simulink model "FourWheelSim_base"  (R2021b)
settings: Solver=ode4  StartTime=0.0  StopTime=100  FixedStep=0.001  EnableMultiTasking=on
values from neighbouring files (symbols this model uses):
  a_f = [1.434106444513048,-3.490394354141787e-04,2.761516722659314,6.000050177239062e+04,2.990012596710455e+03,-1.736376596503330e-04,0.526021936511837]    [VehicleParams20_ver230707.m]
  a_r = a_f    [VehicleParams20_ver230707.m]
  afx_f = [1.736519934348130,-2.903281841026900e-04,2.651682004580759,7.000047010028531e+04,3.270011055825476e+03,-0.001252141095807,1.596836353939939]    [VehicleParams20_ver230707.m]
  afx_r = afx_f    [VehicleParams20_ver230707.m]
  agx_f = [0.230000000000000,2.936116597489246e+04,7.137436879966481e+03,0,0]    [VehicleParams20_ver230707.m]
  agx_r = agx_f    [VehicleParams20_ver230707.m]
  agy_f = [0.852564208514954,3.000069064154418e+04,2.070023877794581e+03,-5.089267464508360e-04,0.519364283925805]    [VehicleParams20_ver230707.m]
  agy_r = agy_f    [VehicleParams20_ver230707.m]
  b_f = [3.436650779629654,1.566044221042620e-05,0.028598122547093,3.408741969645286e+03,5.995144285148312e+03,-1.736376595720277e-04,0.526021936449385]    [VehicleParams20_ver230707.m]
  Brake_Factor = 0.66    [VehicleParams20_ver230707.m]
  Cd = Cd/(40/3.6)^2    (= 0.6885)    [VehicleParams20_ver230707.m]
  CLF = DFf/40/40    (= 0.06)    [VehicleParams20_ver230707.m]
  CLR = DFr/40/40    (= 0.065)    [VehicleParams20_ver230707.m]
  cPiston_Area_F = 2*pi*(0.0254/2)^2    (= 0.00101341495819)    [VehicleParams20_ver230707.m]
  cPiston_Area_R = 2*pi*(0.0254/2)^2    (= 0.00101341495819)    [VehicleParams20_ver230707.m]
  delta = 15.5    [VehicleParams20_ver230707.m]
  df = 1.225    [VehicleParams20_ver230707.m]
  dr = 1.225    [VehicleParams20_ver230707.m]
  eff_Radius_F = (180/2-13.5)/1000    (= 0.0765)    [VehicleParams20_ver230707.m]
  eff_Radius_R = (180/2-13.5)/1000    (= 0.0765)    [VehicleParams20_ver230707.m]
  Fd = 60*2    (= 120)    [VehicleParams20_ver230707.m]
  Frtoe = 0    [VehicleParams20_ver230707.m]
  gear_f = 13.75    [VehicleParams20_ver230707.m]
  gear_r = 13.75    [VehicleParams20_ver230707.m]
  hg = 0.28    [VehicleParams20_ver230707.m]
  HV_voltage = 600    [VehicleParams20_ver230707.m]
  I = 112    [VehicleParams20_ver230707.m]
  ini_v = ini_speed/3.6    (= 10.4166666667)    [VehicleParams20_ver230707.m]
  Kframe = 5.94*10^6    (= 5940000)    [VehicleParams20_ver230707.m]
  kk_f = 2800*180/pi    (= 160428.182637)    [VehicleParams20_ver230707.m]
  kk_r = 4200*180/pi    (= 240642.273955)    [VehicleParams20_ver230707.m]
  krfr = 0.5    [VehicleParams20_ver230707.m]
  l = 1.530    (= 1.53)    [VehicleParams20_ver230707.m]
  lf = l*(1-WBf)    (= 0.7956)    [VehicleParams20_ver230707.m]
  lr = l*WBf    (= 0.7344)    [VehicleParams20_ver230707.m]
  M = 200+60    (= 260)    [VehicleParams20_ver230707.m]
  mu_tire_F = 0.587-0.587+0.55    (= 0.55)    [VehicleParams20_ver230707.m]
  mu_tire_R = 0.587-0.587+0.55    (= 0.55)    [VehicleParams20_ver230707.m]
  Mwf = Iwf/Rwf/Rwf    (= 3.82716814816)    [VehicleParams20_ver230707.m]
  Mwr = Iwr/Rwr/Rwr    (= 3.82716814816)    [VehicleParams20_ver230707.m]
  rcf = 0.000    (= 0)    [VehicleParams20_ver230707.m]
  rch = rcf*WBf+rcr*(1-WBf)    (= 0)    [VehicleParams20_ver230707.m]
  rcr = 0.000    (= 0)    [VehicleParams20_ver230707.m]
  Reartoe = -2    [VehicleParams20_ver230707.m]
  Rr_toe = Reartoe*pi/180    (= -0.0349065850399)    [VehicleParams20_ver230707.m]
  Rwf = 18*(25.4/1000)/2    (= 0.2286)    [VehicleParams20_ver230707.m]
  Rwr = 18*(25.4/1000)/2    (= 0.2286)    [VehicleParams20_ver230707.m]
  T_TireF = TireL_f/V    (= 0.036760000032)    [VehicleParams20_ver230707.m]
  T_TireR = TireL_r/V    (= 0.036760000032)    [VehicleParams20_ver230707.m]
  tspeed = 37.5    [VehicleParams20_ver230707.m]
  WBf = 0.48    [VehicleParams20_ver230707.m]
  zc_f = castrail_Fr/1000    (= 0)    [VehicleParams20_ver230707.m]
  zc_r = castrail_Rr/1000    (= 0)    [VehicleParams20_ver230707.m]
libraries: simulink x25, dspstat3 x1
(part 3 of 4)

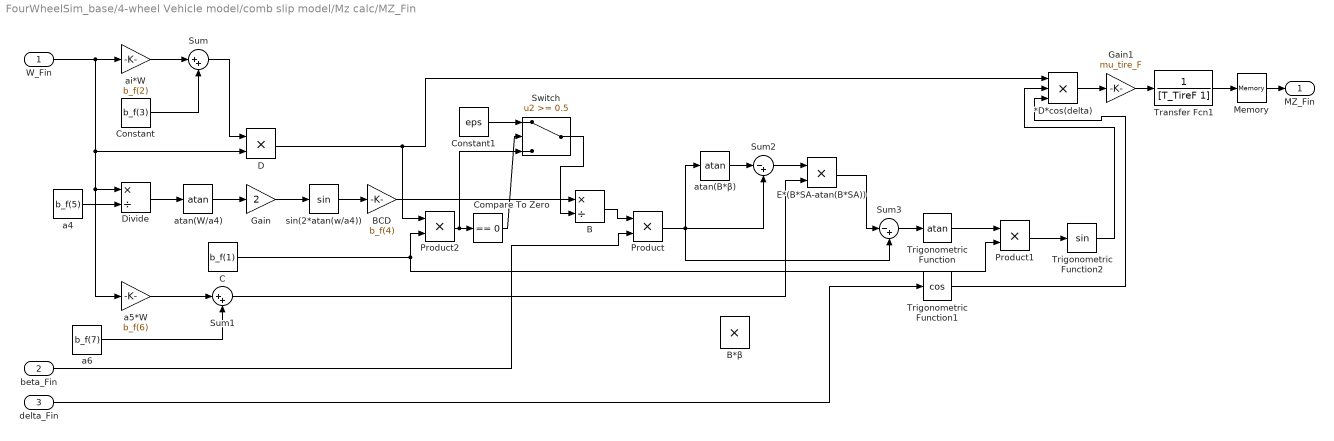
== system FourWheelSim_base/4-wheel Vehicle model/comb slip model/Mz calc/MZ_Fin ==
  W_Fin : Inport
  beta_Fin : Inport  Port=2
  delta_Fin : Inport  Port=3
  *D*cos(delta) : Product  Inputs=3  RndMeth=Zero
  B : Product  Inputs=*/
  B*β : Product  Inputs=**
  BCD : Gain  Gain=b_f(4)
  C : Constant  Value=b_f(1)
  Compare To Zero : simulink/Logic and Bit Operations/Compare To Zero  relop===  OutDataTypeStr=boolean
  Constant : Constant  Value=b_f(3)
  Constant1 : Constant  Value=eps
  D : Product  RndMeth=Zero
  Divide : Product  Inputs=*/
  E*(B*SA-atan(B*SA)) : Product  RndMeth=Zero
  Gain : Gain  Gain=2
  Gain1 : Gain  Gain=mu_tire_F
  Memory : Memory
  Product : Product  RndMeth=Zero
  Product1 : Product  RndMeth=Zero
  Product2 : Product
  Sum : Sum  Inputs=|++
  Sum1 : Sum  Inputs=|++
  Sum2 : Sum  Inputs=|-+
  Sum3 : Sum  Inputs=|-+
  Switch : Switch  Threshold=0.5
  Transfer Fcn1 : TransferFcn  Denominator=[T_TireF 1]
  Trigonometric Function : Trigonometry  Operator=atan
  Trigonometric Function1 : Trigonometry  Operator=cos
  Trigonometric Function2 : Trigonometry
  a4 : Constant  Value=b_f(5)
  a5*W : Gain  Gain=b_f(6)
  a6 : Constant  Value=b_f(7)
  ai*W : Gain  Gain=b_f(2)
  atan(B*β) : Trigonometry  Operator=atan
  atan(W/a4) : Trigonometry  Operator=atan
  sin(2*atan(w/a4)) : Trigonometry
  MZ_Fin : Outport  VectorParamsAs1DForOutWhenUnconnected=off
  wires:
  Constant/1 -> Sum/2
  ai*W/1 -> Sum/1
  Sum/1 -> D/1
  a4/1 -> Divide/2
  Divide/1 -> atan(W/a4)/1
  atan(W/a4)/1 -> Gain/1
  Gain/1 -> sin(2*atan(w/a4))/1
  sin(2*atan(w/a4))/1 -> BCD/1
  BCD/1 -> B/1
  C/1 -> Product1/2, Product2/2
  a5*W/1 -> Sum1/1
  a6/1 -> Sum1/2
  B/1 -> Product/1
  beta_Fin/1 -> Product/2
  Sum1/1 -> E*(B*SA-atan(B*SA))/2
  Sum3/1 -> Trigonometric Function/1
  D/1 -> Product2/1, *D*cos(delta)/1
  Gain1/1 -> Transfer Fcn1/1
  delta_Fin/1 -> Trigonometric Function1/1
  Trigonometric Function1/1 -> *D*cos(delta)/3
  Trigonometric Function/1 -> Product1/1
  Trigonometric Function2/1 -> *D*cos(delta)/2
  Product1/1 -> Trigonometric Function2/1
  W_Fin/1 -> a5*W/1, Divide/1, D/2, ai*W/1
  Product2/1 -> Switch/3, Compare To Zero/1
  Compare To Zero/1 -> Switch/2
  Constant1/1 -> Switch/1
  Switch/1 -> B/2
  *D*cos(delta)/1 -> Gain1/1
  Transfer Fcn1/1 -> Memory/1
  Memory/1 -> MZ_Fin/1
  Product/1 -> Sum2/2, Sum3/2, atan(B*β)/1
  atan(B*β)/1 -> Sum2/1
  Sum2/1 -> E*(B*SA-atan(B*SA))/1
  E*(B*SA-atan(B*SA))/1 -> Sum3/1

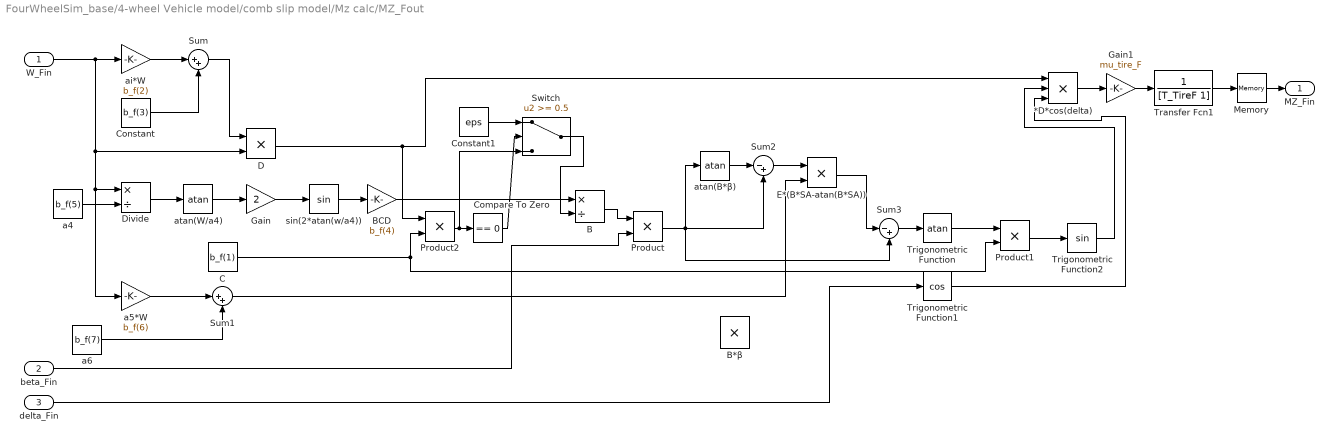
== system FourWheelSim_base/4-wheel Vehicle model/comb slip model/Mz calc/MZ_Fout ==
  W_Fin : Inport
  beta_Fin : Inport  Port=2
  delta_Fin : Inport  Port=3
  *D*cos(delta) : Product  Inputs=3  RndMeth=Zero
  B : Product  Inputs=*/
  B*β : Product  Inputs=**
  BCD : Gain  Gain=b_f(4)
  C : Constant  Value=b_f(1)
  Compare To Zero : simulink/Logic and Bit Operations/Compare To Zero  relop===  OutDataTypeStr=boolean
  Constant : Constant  Value=b_f(3)
  Constant1 : Constant  Value=eps
  D : Product  RndMeth=Zero
  Divide : Product  Inputs=*/
  E*(B*SA-atan(B*SA)) : Product  RndMeth=Zero
  Gain : Gain  Gain=2
  Gain1 : Gain  Gain=mu_tire_F
  Memory : Memory
  Product : Product  RndMeth=Zero
  Product1 : Product  RndMeth=Zero
  Product2 : Product
  Sum : Sum  Inputs=|++
  Sum1 : Sum  Inputs=|++
  Sum2 : Sum  Inputs=|-+
  Sum3 : Sum  Inputs=|-+
  Switch : Switch  Threshold=0.5
  Transfer Fcn1 : TransferFcn  Denominator=[T_TireF 1]
  Trigonometric Function : Trigonometry  Operator=atan
  Trigonometric Function1 : Trigonometry  Operator=cos
  Trigonometric Function2 : Trigonometry
  a4 : Constant  Value=b_f(5)
  a5*W : Gain  Gain=b_f(6)
  a6 : Constant  Value=b_f(7)
  ai*W : Gain  Gain=b_f(2)
  atan(B*β) : Trigonometry  Operator=atan
  atan(W/a4) : Trigonometry  Operator=atan
  sin(2*atan(w/a4)) : Trigonometry
  MZ_Fin : Outport  VectorParamsAs1DForOutWhenUnconnected=off
  wires:
  Constant/1 -> Sum/2
  ai*W/1 -> Sum/1
  Sum/1 -> D/1
  a4/1 -> Divide/2
  Divide/1 -> atan(W/a4)/1
  atan(W/a4)/1 -> Gain/1
  Gain/1 -> sin(2*atan(w/a4))/1
  sin(2*atan(w/a4))/1 -> BCD/1
  BCD/1 -> B/1
  C/1 -> Product1/2, Product2/2
  a5*W/1 -> Sum1/1
  a6/1 -> Sum1/2
  B/1 -> Product/1
  beta_Fin/1 -> Product/2
  Sum1/1 -> E*(B*SA-atan(B*SA))/2
  Sum3/1 -> Trigonometric Function/1
  D/1 -> Product2/1, *D*cos(delta)/1
  Gain1/1 -> Transfer Fcn1/1
  delta_Fin/1 -> Trigonometric Function1/1
  Trigonometric Function1/1 -> *D*cos(delta)/3
  Trigonometric Function/1 -> Product1/1
  Trigonometric Function2/1 -> *D*cos(delta)/2
  Product1/1 -> Trigonometric Function2/1
  W_Fin/1 -> a5*W/1, Divide/1, D/2, ai*W/1
  Product2/1 -> Switch/3, Compare To Zero/1
  Compare To Zero/1 -> Switch/2
  Constant1/1 -> Switch/1
  Switch/1 -> B/2
  *D*cos(delta)/1 -> Gain1/1
  Transfer Fcn1/1 -> Memory/1
  Memory/1 -> MZ_Fin/1
  Product/1 -> Sum2/2, Sum3/2, atan(B*β)/1
  atan(B*β)/1 -> Sum2/1
  Sum2/1 -> E*(B*SA-atan(B*SA))/1
  E*(B*SA-atan(B*SA))/1 -> Sum3/1

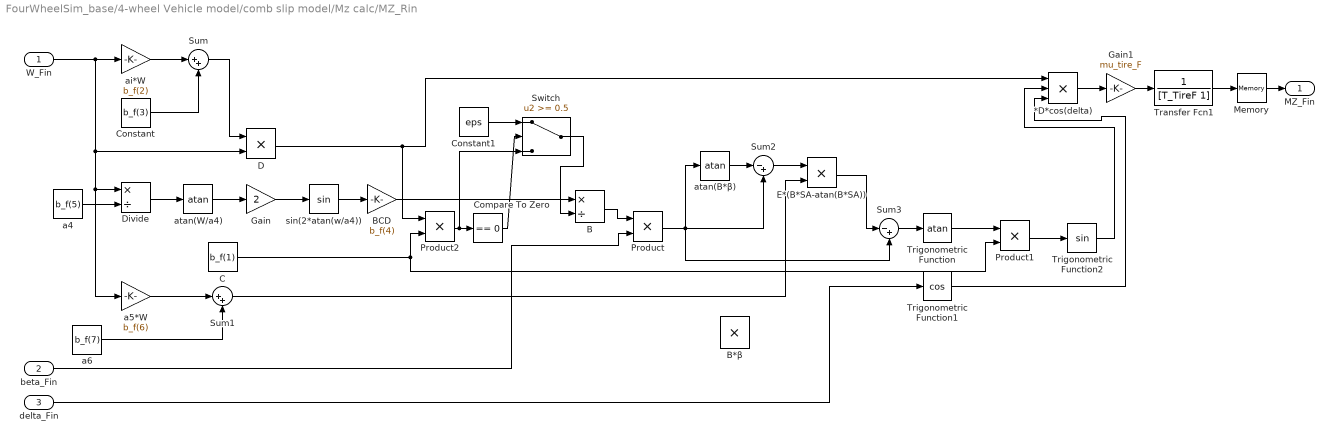
== system FourWheelSim_base/4-wheel Vehicle model/comb slip model/Mz calc/MZ_Rin ==
  W_Fin : Inport
  beta_Fin : Inport  Port=2
  delta_Fin : Inport  Port=3
  *D*cos(delta) : Product  Inputs=3  RndMeth=Zero
  B : Product  Inputs=*/
  B*β : Product  Inputs=**
  BCD : Gain  Gain=b_f(4)
  C : Constant  Value=b_f(1)
  Compare To Zero : simulink/Logic and Bit Operations/Compare To Zero  relop===  OutDataTypeStr=boolean
  Constant : Constant  Value=b_f(3)
  Constant1 : Constant  Value=eps
  D : Product  RndMeth=Zero
  Divide : Product  Inputs=*/
  E*(B*SA-atan(B*SA)) : Product  RndMeth=Zero
  Gain : Gain  Gain=2
  Gain1 : Gain  Gain=mu_tire_F
  Memory : Memory
  Product : Product  RndMeth=Zero
  Product1 : Product  RndMeth=Zero
  Product2 : Product
  Sum : Sum  Inputs=|++
  Sum1 : Sum  Inputs=|++
  Sum2 : Sum  Inputs=|-+
  Sum3 : Sum  Inputs=|-+
  Switch : Switch  Threshold=0.5
  Transfer Fcn1 : TransferFcn  Denominator=[T_TireF 1]
  Trigonometric Function : Trigonometry  Operator=atan
  Trigonometric Function1 : Trigonometry  Operator=cos
  Trigonometric Function2 : Trigonometry
  a4 : Constant  Value=b_f(5)
  a5*W : Gain  Gain=b_f(6)
  a6 : Constant  Value=b_f(7)
  ai*W : Gain  Gain=b_f(2)
  atan(B*β) : Trigonometry  Operator=atan
  atan(W/a4) : Trigonometry  Operator=atan
  sin(2*atan(w/a4)) : Trigonometry
  MZ_Fin : Outport  VectorParamsAs1DForOutWhenUnconnected=off
  wires:
  Constant/1 -> Sum/2
  ai*W/1 -> Sum/1
  Sum/1 -> D/1
  a4/1 -> Divide/2
  Divide/1 -> atan(W/a4)/1
  atan(W/a4)/1 -> Gain/1
  Gain/1 -> sin(2*atan(w/a4))/1
  sin(2*atan(w/a4))/1 -> BCD/1
  BCD/1 -> B/1
  C/1 -> Product1/2, Product2/2
  a5*W/1 -> Sum1/1
  a6/1 -> Sum1/2
  B/1 -> Product/1
  beta_Fin/1 -> Product/2
  Sum1/1 -> E*(B*SA-atan(B*SA))/2
  Sum3/1 -> Trigonometric Function/1
  D/1 -> Product2/1, *D*cos(delta)/1
  Gain1/1 -> Transfer Fcn1/1
  delta_Fin/1 -> Trigonometric Function1/1
  Trigonometric Function1/1 -> *D*cos(delta)/3
  Trigonometric Function/1 -> Product1/1
  Trigonometric Function2/1 -> *D*cos(delta)/2
  Product1/1 -> Trigonometric Function2/1
  W_Fin/1 -> a5*W/1, Divide/1, D/2, ai*W/1
  Product2/1 -> Switch/3, Compare To Zero/1
  Compare To Zero/1 -> Switch/2
  Constant1/1 -> Switch/1
  Switch/1 -> B/2
  *D*cos(delta)/1 -> Gain1/1
  Transfer Fcn1/1 -> Memory/1
  Memory/1 -> MZ_Fin/1
  Product/1 -> Sum2/2, Sum3/2, atan(B*β)/1
  atan(B*β)/1 -> Sum2/1
  Sum2/1 -> E*(B*SA-atan(B*SA))/1
  E*(B*SA-atan(B*SA))/1 -> Sum3/1

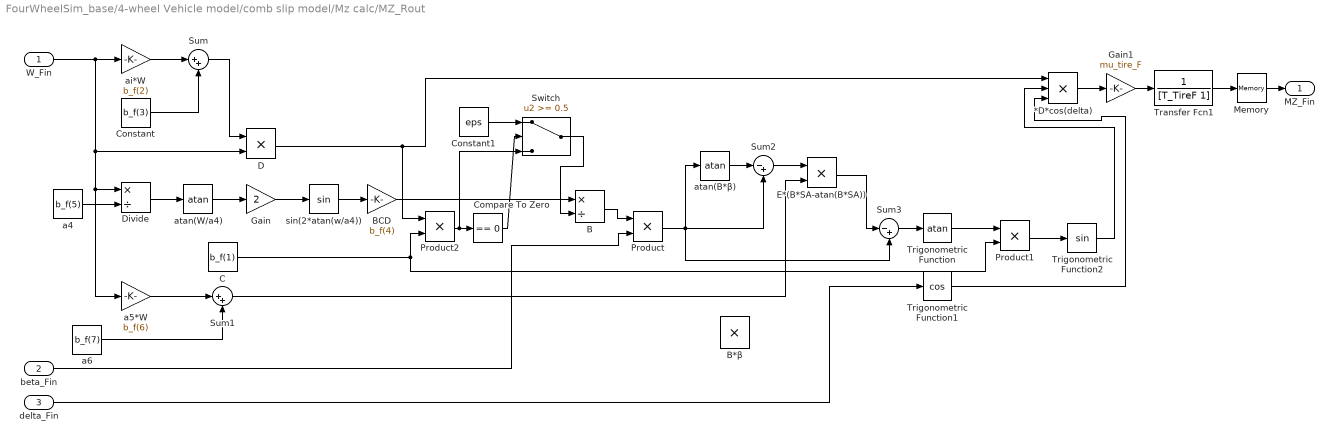
== system FourWheelSim_base/4-wheel Vehicle model/comb slip model/Mz calc/MZ_Rout ==
  W_Fin : Inport
  beta_Fin : Inport  Port=2
  delta_Fin : Inport  Port=3
  *D*cos(delta) : Product  Inputs=3  RndMeth=Zero
  B : Product  Inputs=*/
  B*β : Product  Inputs=**
  BCD : Gain  Gain=b_f(4)
  C : Constant  Value=b_f(1)
  Compare To Zero : simulink/Logic and Bit Operations/Compare To Zero  relop===  OutDataTypeStr=boolean
  Constant : Constant  Value=b_f(3)
  Constant1 : Constant  Value=eps
  D : Product  RndMeth=Zero
  Divide : Product  Inputs=*/
  E*(B*SA-atan(B*SA)) : Product  RndMeth=Zero
  Gain : Gain  Gain=2
  Gain1 : Gain  Gain=mu_tire_F
  Memory : Memory
  Product : Product  RndMeth=Zero
  Product1 : Product  RndMeth=Zero
  Product2 : Product
  Sum : Sum  Inputs=|++
  Sum1 : Sum  Inputs=|++
  Sum2 : Sum  Inputs=|-+
  Sum3 : Sum  Inputs=|-+
  Switch : Switch  Threshold=0.5
  Transfer Fcn1 : TransferFcn  Denominator=[T_TireF 1]
  Trigonometric Function : Trigonometry  Operator=atan
  Trigonometric Function1 : Trigonometry  Operator=cos
  Trigonometric Function2 : Trigonometry
  a4 : Constant  Value=b_f(5)
  a5*W : Gain  Gain=b_f(6)
  a6 : Constant  Value=b_f(7)
  ai*W : Gain  Gain=b_f(2)
  atan(B*β) : Trigonometry  Operator=atan
  atan(W/a4) : Trigonometry  Operator=atan
  sin(2*atan(w/a4)) : Trigonometry
  MZ_Fin : Outport  VectorParamsAs1DForOutWhenUnconnected=off
  wires:
  Constant/1 -> Sum/2
  ai*W/1 -> Sum/1
  Sum/1 -> D/1
  a4/1 -> Divide/2
  Divide/1 -> atan(W/a4)/1
  atan(W/a4)/1 -> Gain/1
  Gain/1 -> sin(2*atan(w/a4))/1
  sin(2*atan(w/a4))/1 -> BCD/1
  BCD/1 -> B/1
  C/1 -> Product1/2, Product2/2
  a5*W/1 -> Sum1/1
  a6/1 -> Sum1/2
  B/1 -> Product/1
  beta_Fin/1 -> Product/2
  Sum1/1 -> E*(B*SA-atan(B*SA))/2
  Sum3/1 -> Trigonometric Function/1
  D/1 -> Product2/1, *D*cos(delta)/1
  Gain1/1 -> Transfer Fcn1/1
  delta_Fin/1 -> Trigonometric Function1/1
  Trigonometric Function1/1 -> *D*cos(delta)/3
  Trigonometric Function/1 -> Product1/1
  Trigonometric Function2/1 -> *D*cos(delta)/2
  Product1/1 -> Trigonometric Function2/1
  W_Fin/1 -> a5*W/1, Divide/1, D/2, ai*W/1
  Product2/1 -> Switch/3, Compare To Zero/1
  Compare To Zero/1 -> Switch/2
  Constant1/1 -> Switch/1
  Switch/1 -> B/2
  *D*cos(delta)/1 -> Gain1/1
  Transfer Fcn1/1 -> Memory/1
  Memory/1 -> MZ_Fin/1
  Product/1 -> Sum2/2, Sum3/2, atan(B*β)/1
  atan(B*β)/1 -> Sum2/1
  Sum2/1 -> E*(B*SA-atan(B*SA))/1
  E*(B*SA-atan(B*SA))/1 -> Sum3/1

== system FourWheelSim_base/4-wheel Vehicle model/comb slip model/comb Fx calc/Force_Fin_comb_FX ==
  W_Fin : Inport
  beta_Fin : Inport  Port=2
  slip rate : Inport  Port=3
  *D : Product  RndMeth=Zero
  B : Product  Inputs=*/
  BCD : Gain  Gain=agx_f(2)
  C : Constant  Value=agx_f(1)
  Compare To Zero : simulink/Logic and Bit Operations/Compare To Zero  relop===  OutDataTypeStr=boolean
  Constant1 : Constant  Value=eps
  Divide : Product  Inputs=*/
  E*(B*SA-atan(B*SA)) : Product  RndMeth=Zero
  Gain : Gain  Gain=2
  Gain1 : Gain  Gain=mu_tire_F
  Product : Product  RndMeth=Zero
  Product1 : Product  RndMeth=Zero
  Product2 : Product
  Scope : Scope
  Sum1 : Sum  Inputs=|++
  Sum2 : Sum  Inputs=|-+
  Sum3 : Sum  Inputs=|-+
  Switch : Switch  Threshold=0.5
  Tire Force : Subsystem
  Trigonometric Function : Trigonometry  Operator=atan
  Trigonometric Function2 : Trigonometry  Operator=cos
  a4 : Constant  Value=agx_f(3)
  a5*W : Gain  Gain=agy_f(4)
  a6 : Constant  Value=agx_f(5)
  atan(B*β) : Trigonometry  Operator=atan
  atan(W/a4) : Trigonometry  Operator=atan
  sin(2*atan(w/a4)) : Trigonometry
  Force_Fin : Outport  VectorParamsAs1DForOutWhenUnconnected=off
  wires:
  a4/1 -> Divide/2
  Divide/1 -> atan(W/a4)/1
  atan(W/a4)/1 -> Gain/1
  Gain/1 -> sin(2*atan(w/a4))/1
  sin(2*atan(w/a4))/1 -> BCD/1
  C/1 -> Product1/2, Product2/2
  a5*W/1 -> Sum1/1
  a6/1 -> Sum1/2
  B/1 -> Product/1
  Sum1/1 -> E*(B*SA-atan(B*SA))/2
  Sum3/1 -> Trigonometric Function/1
  Trigonometric Function/1 -> Product1/1
  Trigonometric Function2/1 -> *D/2
  Product1/1 -> Trigonometric Function2/1
  W_Fin/1 -> Tire Force/1(Load), Scope/1, a5*W/1, Divide/1
  *D/1 -> Gain1/1
  Gain1/1 -> Force_Fin/1
  Product/1 -> Sum2/2, Sum3/2, atan(B*β)/1
  atan(B*β)/1 -> Sum2/1
  Sum2/1 -> E*(B*SA-atan(B*SA))/1
  E*(B*SA-atan(B*SA))/1 -> Sum3/1
  Tire Force/1(Force_Rear) -> Product2/1, *D/1
  Product2/1 -> Switch/3, Compare To Zero/1
  Constant1/1 -> Switch/1
  Switch/1 -> B/2
  Compare To Zero/1 -> Switch/2
  BCD/1 -> B/1
  slip rate/1 -> Tire Force/2(Slip Rate)
  beta_Fin/1 -> Product/2

== system FourWheelSim_base/4-wheel Vehicle model/comb slip model/comb Fx calc/Force_Fout_comb_FX ==
  W_Fout : Inport
  beta_Fout : Inport  Port=2
  slip rate : Inport  Port=3
  *D : Product  RndMeth=Zero
  B : Product  Inputs=*/
  BCD : Gain  Gain=agx_f(2)
  C : Constant  Value=agx_f(1)
  Compare To Zero : simulink/Logic and Bit Operations/Compare To Zero  relop===  OutDataTypeStr=boolean
  Constant1 : Constant  Value=eps
  Divide : Product  Inputs=*/
  E*(B*SA-atan(B*SA)) : Product  RndMeth=Zero
  Gain : Gain  Gain=2
  Gain1 : Gain  Gain=mu_tire_F
  Product : Product  RndMeth=Zero
  Product1 : Product  RndMeth=Zero
  Product2 : Product
  Sum1 : Sum  Inputs=|++
  Sum2 : Sum  Inputs=|-+
  Sum3 : Sum  Inputs=|-+
  Switch : Switch  Threshold=0.5
  Tire Force : Subsystem
  Trigonometric Function : Trigonometry  Operator=atan
  Trigonometric Function2 : Trigonometry  Operator=cos
  a4 : Constant  Value=agx_f(3)
  a5*W : Gain  Gain=agy_f(4)
  a6 : Constant  Value=agx_f(5)
  atan(B*β) : Trigonometry  Operator=atan
  atan(W/a4) : Trigonometry  Operator=atan
  sin(2*atan(w/a4)) : Trigonometry
  Force_Fout : Outport  VectorParamsAs1DForOutWhenUnconnected=off
  wires:
  a4/1 -> Divide/2
  Divide/1 -> atan(W/a4)/1
  atan(W/a4)/1 -> Gain/1
  Gain/1 -> sin(2*atan(w/a4))/1
  sin(2*atan(w/a4))/1 -> BCD/1
  C/1 -> Product1/2, Product2/2
  a5*W/1 -> Sum1/1
  a6/1 -> Sum1/2
  B/1 -> Product/1
  Sum1/1 -> E*(B*SA-atan(B*SA))/2
  Sum3/1 -> Trigonometric Function/1
  Trigonometric Function/1 -> Product1/1
  Trigonometric Function2/1 -> *D/2
  Product1/1 -> Trigonometric Function2/1
  W_Fout/1 -> Tire Force/1(Load), a5*W/1, Divide/1
  *D/1 -> Gain1/1
  Product/1 -> Sum2/2, Sum3/2, atan(B*β)/1
  atan(B*β)/1 -> Sum2/1
  Sum2/1 -> E*(B*SA-atan(B*SA))/1
  E*(B*SA-atan(B*SA))/1 -> Sum3/1
  Tire Force/1(Force_Rear) -> Product2/1, *D/1
  Product2/1 -> Switch/3, Compare To Zero/1
  Constant1/1 -> Switch/1
  Switch/1 -> B/2
  Compare To Zero/1 -> Switch/2
  BCD/1 -> B/1
  slip rate/1 -> Tire Force/2(Slip Rate)
  beta_Fout/1 -> Product/2
  Gain1/1 -> Force_Fout/1

== system FourWheelSim_base/4-wheel Vehicle model/comb slip model/comb Fx calc/Force_Rin_comb_FX ==
  W_Rin : Inport
  beta_Rin : Inport  Port=2
  slip rate : Inport  Port=3
  *D : Product  RndMeth=Zero
  B : Product  Inputs=*/
  BCD : Gain  Gain=agx_r(2)
  C : Constant  Value=agx_r(1)
  Compare To Zero : simulink/Logic and Bit Operations/Compare To Zero  relop===  OutDataTypeStr=boolean
  Constant1 : Constant  Value=eps
  Divide : Product  Inputs=*/
  E*(B*SA-atan(B*SA)) : Product  RndMeth=Zero
  Gain : Gain  Gain=2
  Gain1 : Gain  Gain=mu_tire_R
  Product : Product  RndMeth=Zero
  Product1 : Product  RndMeth=Zero
  Product2 : Product
  Sum1 : Sum  Inputs=|++
  Sum2 : Sum  Inputs=|-+
  Sum3 : Sum  Inputs=|-+
  Switch : Switch  Threshold=0.5
  Tire Force : Subsystem
  Trigonometric Function : Trigonometry  Operator=atan
  Trigonometric Function2 : Trigonometry  Operator=cos
  a4 : Constant  Value=agx_r(3)
  a5*W : Gain  Gain=agy_r(4)
  a6 : Constant  Value=agx_r(5)
  atan(B*β) : Trigonometry  Operator=atan
  atan(W/a4) : Trigonometry  Operator=atan
  sin(2*atan(w/a4)) : Trigonometry
  Force_Rin : Outport  VectorParamsAs1DForOutWhenUnconnected=off
  wires:
  a4/1 -> Divide/2
  Divide/1 -> atan(W/a4)/1
  atan(W/a4)/1 -> Gain/1
  Gain/1 -> sin(2*atan(w/a4))/1
  sin(2*atan(w/a4))/1 -> BCD/1
  C/1 -> Product1/2, Product2/2
  a5*W/1 -> Sum1/1
  a6/1 -> Sum1/2
  B/1 -> Product/1
  Sum1/1 -> E*(B*SA-atan(B*SA))/2
  Sum3/1 -> Trigonometric Function/1
  Trigonometric Function/1 -> Product1/1
  Trigonometric Function2/1 -> *D/2
  Product1/1 -> Trigonometric Function2/1
  W_Rin/1 -> Tire Force/1(Load), a5*W/1, Divide/1
  Product/1 -> Sum2/2, Sum3/2, atan(B*β)/1
  atan(B*β)/1 -> Sum2/1
  Sum2/1 -> E*(B*SA-atan(B*SA))/1
  E*(B*SA-atan(B*SA))/1 -> Sum3/1
  Tire Force/1(Force_Rear) -> Product2/1, *D/1
  Product2/1 -> Switch/3, Compare To Zero/1
  Constant1/1 -> Switch/1
  Switch/1 -> B/2
  Compare To Zero/1 -> Switch/2
  BCD/1 -> B/1
  slip rate/1 -> Tire Force/2(Slip Rate)
  beta_Rin/1 -> Product/2
  Gain1/1 -> Force_Rin/1
  *D/1 -> Gain1/1

== system FourWheelSim_base/4-wheel Vehicle model/comb slip model/comb Fx calc/Force_Rout_comb1_FX ==
  W_Rout : Inport
  beta_Rout : Inport  Port=2
  slip rate : Inport  Port=3
  *D : Product  RndMeth=Zero
  B : Product  Inputs=*/
  BCD : Gain  Gain=agx_r(2)
  C : Constant  Value=agx_r(1)
  Compare To Zero : simulink/Logic and Bit Operations/Compare To Zero  relop===  OutDataTypeStr=boolean
  Constant1 : Constant  Value=eps
  Divide : Product  Inputs=*/
  E*(B*SA-atan(B*SA)) : Product  RndMeth=Zero
  Gain : Gain  Gain=2
  Gain1 : Gain  Gain=mu_tire_R
  Product : Product  RndMeth=Zero
  Product1 : Product  RndMeth=Zero
  Product2 : Product
  Scope : Scope
  Sum1 : Sum  Inputs=|++
  Sum2 : Sum  Inputs=|-+
  Sum3 : Sum  Inputs=|-+
  Switch : Switch  Threshold=0.5
  Tire Force : Subsystem
  Trigonometric Function : Trigonometry  Operator=atan
  Trigonometric Function2 : Trigonometry  Operator=cos
  a4 : Constant  Value=agx_r(3)
  a5*W : Gain  Gain=agy_r(4)
  a6 : Constant  Value=agx_r(5)
  atan(B*β) : Trigonometry  Operator=atan
  atan(W/a4) : Trigonometry  Operator=atan
  sin(2*atan(w/a4)) : Trigonometry
  Force_Rin : Outport  VectorParamsAs1DForOutWhenUnconnected=off
  wires:
  a4/1 -> Divide/2
  Divide/1 -> Scope/1, atan(W/a4)/1
  atan(W/a4)/1 -> Gain/1
  Gain/1 -> sin(2*atan(w/a4))/1
  sin(2*atan(w/a4))/1 -> BCD/1
  C/1 -> Product1/2, Product2/2
  a5*W/1 -> Sum1/1
  a6/1 -> Sum1/2
  B/1 -> Product/1
  Sum1/1 -> E*(B*SA-atan(B*SA))/2
  Sum3/1 -> Trigonometric Function/1
  Trigonometric Function/1 -> Product1/1
  Trigonometric Function2/1 -> *D/2
  Product1/1 -> Trigonometric Function2/1
  W_Rout/1 -> Tire Force/1(Load), a5*W/1, Divide/1
  Product/1 -> Sum2/2, Sum3/2, atan(B*β)/1
  atan(B*β)/1 -> Sum2/1
  Sum2/1 -> E*(B*SA-atan(B*SA))/1
  E*(B*SA-atan(B*SA))/1 -> Sum3/1
  Tire Force/1(Force_Rear) -> Product2/1, *D/1
  Product2/1 -> Switch/3, Compare To Zero/1
  Constant1/1 -> Switch/1
  Switch/1 -> B/2
  Compare To Zero/1 -> Switch/2
  BCD/1 -> B/1
  slip rate/1 -> Tire Force/2(Slip Rate)
  beta_Rout/1 -> Product/2
  Gain1/1 -> Force_Rin/1
  *D/1 -> Gain1/1

== system FourWheelSim_base/4-wheel Vehicle model/comb slip model/comb Fy calc/Force_Fin_comb_FY ==
  W_Fin : Inport
  beta_Fin : Inport  Port=2
  slip rate : Inport  Port=3
  *D : Product  RndMeth=Zero
  B : Product  Inputs=*/
  BCD : Gain  Gain=agy_f(2)
  C : Constant  Value=agy_f(1)
  Compare To Zero : simulink/Logic and Bit Operations/Compare To Zero  relop===  OutDataTypeStr=boolean
  Constant1 : Constant  Value=eps
  Divide : Product  Inputs=*/
  E*(B*SA-atan(B*SA)) : Product  RndMeth=Zero
  Force_Fin_Pure : Subsystem
  Gain : Gain  Gain=2
  Gain1 : Gain  Gain=-mu_tire_F
  Product : Product  RndMeth=Zero
  Product1 : Product  RndMeth=Zero
  Product2 : Product
  Sum1 : Sum  Inputs=|++
  Sum2 : Sum  Inputs=|-+
  Sum3 : Sum  Inputs=|-+
  Switch : Switch  Threshold=0.5
  Transfer Fcn1 : TransferFcn  Denominator=[T_TireF 1]
  Trigonometric Function : Trigonometry  Operator=atan
  Trigonometric Function2 : Trigonometry  Operator=cos
  a4 : Constant  Value=agy_f(3)
  a5*W : Gain  Gain=agy_f(4)
  a6 : Constant  Value=agy_f(5)
  atan(B*β) : Trigonometry  Operator=atan
  atan(W/a4) : Trigonometry  Operator=atan
  sin(2*atan(w/a4)) : Trigonometry
  Force_Fin : Outport  VectorParamsAs1DForOutWhenUnconnected=off
  wires:
  a4/1 -> Divide/2
  Divide/1 -> atan(W/a4)/1
  atan(W/a4)/1 -> Gain/1
  Gain/1 -> sin(2*atan(w/a4))/1
  sin(2*atan(w/a4))/1 -> BCD/1
  C/1 -> Product1/2, Product2/2
  a5*W/1 -> Sum1/1
  a6/1 -> Sum1/2
  B/1 -> Product/1
  beta_Fin/1 -> Force_Fin_Pure/2(beta_Fin)
  Sum1/1 -> E*(B*SA-atan(B*SA))/2
  Sum3/1 -> Trigonometric Function/1
  Gain1/1 -> Transfer Fcn1/1
  Trigonometric Function/1 -> Product1/1
  Trigonometric Function2/1 -> *D/2
  Product1/1 -> Trigonometric Function2/1
  W_Fin/1 -> Force_Fin_Pure/1(W_Fin), a5*W/1, Divide/1
  *D/1 -> Gain1/1
  Transfer Fcn1/1 -> Force_Fin/1
  Product/1 -> Sum2/2, Sum3/2, atan(B*β)/1
  atan(B*β)/1 -> Sum2/1
  Sum2/1 -> E*(B*SA-atan(B*SA))/1
  E*(B*SA-atan(B*SA))/1 -> Sum3/1
  Force_Fin_Pure/1(Force_Fin_Pure) -> Product2/1, *D/1
  slip rate/1 -> Product/2
  Product2/1 -> Switch/3, Compare To Zero/1
  Constant1/1 -> Switch/1
  Switch/1 -> B/2
  Compare To Zero/1 -> Switch/2
  BCD/1 -> B/1

== system FourWheelSim_base/4-wheel Vehicle model/comb slip model/comb Fy calc/Force_Fout_comb_FY ==
  W_Fin : Inport
  beta_Fin : Inport  Port=2
  slip rate : Inport  Port=3
  *D : Product  RndMeth=Zero
  B : Product  Inputs=*/
  BCD : Gain  Gain=agy_f(2)
  C : Constant  Value=agy_f(1)
  Compare To Zero : simulink/Logic and Bit Operations/Compare To Zero  relop===  OutDataTypeStr=boolean
  Constant1 : Constant  Value=eps
  Divide : Product  Inputs=*/
  E*(B*SA-atan(B*SA)) : Product  RndMeth=Zero
  Force_Fout_Pure : Subsystem
  Gain : Gain  Gain=2
  Gain1 : Gain  Gain=-mu_tire_F
  Product : Product  RndMeth=Zero
  Product1 : Product  RndMeth=Zero
  Product2 : Product
  Sum1 : Sum  Inputs=|++
  Sum2 : Sum  Inputs=|-+
  Sum3 : Sum  Inputs=|-+
  Switch : Switch  Threshold=0.5
  Transfer Fcn1 : TransferFcn  Denominator=[T_TireF 1]
  Trigonometric Function : Trigonometry  Operator=atan
  Trigonometric Function2 : Trigonometry  Operator=cos
  a4 : Constant  Value=agy_f(3)
  a5*W : Gain  Gain=agy_f(4)
  a6 : Constant  Value=agy_f(5)
  atan(B*β) : Trigonometry  Operator=atan
  atan(W/a4) : Trigonometry  Operator=atan
  sin(2*atan(w/a4)) : Trigonometry
  Force_Fout : Outport  VectorParamsAs1DForOutWhenUnconnected=off
  wires:
  a4/1 -> Divide/2
  Divide/1 -> atan(W/a4)/1
  atan(W/a4)/1 -> Gain/1
  Gain/1 -> sin(2*atan(w/a4))/1
  sin(2*atan(w/a4))/1 -> BCD/1
  C/1 -> Product1/2, Product2/2
  a5*W/1 -> Sum1/1
  a6/1 -> Sum1/2
  B/1 -> Product/1
  beta_Fin/1 -> Force_Fout_Pure/2(beta_Fin)
  Sum1/1 -> E*(B*SA-atan(B*SA))/2
  Sum3/1 -> Trigonometric Function/1
  Gain1/1 -> Transfer Fcn1/1
  Trigonometric Function/1 -> Product1/1
  Trigonometric Function2/1 -> *D/2
  Product1/1 -> Trigonometric Function2/1
  W_Fin/1 -> Force_Fout_Pure/1(W_Fin), a5*W/1, Divide/1
  *D/1 -> Gain1/1
  Transfer Fcn1/1 -> Force_Fout/1
  Product/1 -> Sum2/2, Sum3/2, atan(B*β)/1
  atan(B*β)/1 -> Sum2/1
  Sum2/1 -> E*(B*SA-atan(B*SA))/1
  E*(B*SA-atan(B*SA))/1 -> Sum3/1
  Force_Fout_Pure/1(Force_Fout_Pure) -> Product2/1, *D/1
  slip rate/1 -> Product/2
  Product2/1 -> Switch/3, Compare To Zero/1
  Constant1/1 -> Switch/1
  Switch/1 -> B/2
  Compare To Zero/1 -> Switch/2
  BCD/1 -> B/1

== system FourWheelSim_base/4-wheel Vehicle model/comb slip model/comb Fy calc/Force_Rin_comb_FY ==
  W_Fin : Inport
  beta_Fin : Inport  Port=2
  slip rate : Inport  Port=3
  *D : Product  RndMeth=Zero
  B : Product  Inputs=*/
  BCD : Gain  Gain=agy_r(2)
  C : Constant  Value=agy_r(1)
  Compare To Zero : simulink/Logic and Bit Operations/Compare To Zero  relop===  OutDataTypeStr=boolean
  Constant1 : Constant  Value=eps
  Divide : Product  Inputs=*/
  E*(B*SA-atan(B*SA)) : Product  RndMeth=Zero
  "Force_Rin_Pure " : Subsystem
  Gain : Gain  Gain=2
  Gain1 : Gain  Gain=-mu_tire_R
  Product : Product  RndMeth=Zero
  Product1 : Product  RndMeth=Zero
  Product2 : Product
  Sum1 : Sum  Inputs=|++
  Sum2 : Sum  Inputs=|-+
  Sum3 : Sum  Inputs=|-+
  Switch : Switch  Threshold=0.5
  Transfer Fcn1 : TransferFcn  Denominator=[T_TireR 1]
  Trigonometric Function : Trigonometry  Operator=atan
  Trigonometric Function2 : Trigonometry  Operator=cos
  a4 : Constant  Value=agy_r(3)
  a5*W : Gain  Gain=agy_r(4)
  a6 : Constant  Value=agy_r(5)
  atan(B*β) : Trigonometry  Operator=atan
  atan(W/a4) : Trigonometry  Operator=atan
  sin(2*atan(w/a4)) : Trigonometry
  Force_Rin : Outport  VectorParamsAs1DForOutWhenUnconnected=off
  wires:
  a4/1 -> Divide/2
  Divide/1 -> atan(W/a4)/1
  atan(W/a4)/1 -> Gain/1
  Gain/1 -> sin(2*atan(w/a4))/1
  sin(2*atan(w/a4))/1 -> BCD/1
  C/1 -> Product1/2, Product2/2
  a5*W/1 -> Sum1/1
  a6/1 -> Sum1/2
  B/1 -> Product/1
  beta_Fin/1 -> "Force_Rin_Pure "/2(beta_Fin)
  Sum1/1 -> E*(B*SA-atan(B*SA))/2
  Sum3/1 -> Trigonometric Function/1
  Gain1/1 -> Transfer Fcn1/1
  Trigonometric Function/1 -> Product1/1
  Trigonometric Function2/1 -> *D/2
  Product1/1 -> Trigonometric Function2/1
  W_Fin/1 -> "Force_Rin_Pure "/1(W_Fin), a5*W/1, Divide/1
  *D/1 -> Gain1/1
  Transfer Fcn1/1 -> Force_Rin/1
  Product/1 -> Sum2/2, Sum3/2, atan(B*β)/1
  atan(B*β)/1 -> Sum2/1
  Sum2/1 -> E*(B*SA-atan(B*SA))/1
  E*(B*SA-atan(B*SA))/1 -> Sum3/1
  "Force_Rin_Pure "/1(Force_Rin_Pure) -> Product2/1, *D/1
  slip rate/1 -> Product/2
  Product2/1 -> Switch/3, Compare To Zero/1
  Constant1/1 -> Switch/1
  Switch/1 -> B/2
  Compare To Zero/1 -> Switch/2
  BCD/1 -> B/1

== system FourWheelSim_base/4-wheel Vehicle model/comb slip model/comb Fy calc/Force_Rout_comb_FY ==
  W_Fin : Inport
  beta_Fin : Inport  Port=2
  slip rate : Inport  Port=3
  *D : Product  RndMeth=Zero
  B : Product  Inputs=*/
  BCD : Gain  Gain=agy_r(2)
  C : Constant  Value=agy_r(1)
  Compare To Zero : simulink/Logic and Bit Operations/Compare To Zero  relop===  OutDataTypeStr=boolean
  Constant1 : Constant  Value=eps
  Divide : Product  Inputs=*/
  E*(B*SA-atan(B*SA)) : Product  RndMeth=Zero
  "Force_Rout_Pure " : Subsystem
  Gain : Gain  Gain=2
  Gain1 : Gain  Gain=-mu_tire_R
  Product : Product  RndMeth=Zero
  Product1 : Product  RndMeth=Zero
  Product2 : Product
  Sum1 : Sum  Inputs=|++
  Sum2 : Sum  Inputs=|-+
  Sum3 : Sum  Inputs=|-+
  Switch : Switch  Threshold=0.5
  Transfer Fcn1 : TransferFcn  Denominator=[T_TireR 1]
  Trigonometric Function : Trigonometry  Operator=atan
  Trigonometric Function2 : Trigonometry  Operator=cos
  a4 : Constant  Value=agy_r(3)
  a5*W : Gain  Gain=agy_r(4)
  a6 : Constant  Value=agy_r(5)
  atan(B*β) : Trigonometry  Operator=atan
  atan(W/a4) : Trigonometry  Operator=atan
  sin(2*atan(w/a4)) : Trigonometry
  Force_Rout : Outport  VectorParamsAs1DForOutWhenUnconnected=off
  wires:
  a4/1 -> Divide/2
  Divide/1 -> atan(W/a4)/1
  atan(W/a4)/1 -> Gain/1
  Gain/1 -> sin(2*atan(w/a4))/1
  sin(2*atan(w/a4))/1 -> BCD/1
  C/1 -> Product1/2, Product2/2
  a5*W/1 -> Sum1/1
  a6/1 -> Sum1/2
  B/1 -> Product/1
  beta_Fin/1 -> "Force_Rout_Pure "/2(beta_Fin)
  Sum1/1 -> E*(B*SA-atan(B*SA))/2
  Sum3/1 -> Trigonometric Function/1
  Gain1/1 -> Transfer Fcn1/1
  Trigonometric Function/1 -> Product1/1
  Trigonometric Function2/1 -> *D/2
  Product1/1 -> Trigonometric Function2/1
  W_Fin/1 -> "Force_Rout_Pure "/1(W_Fin), a5*W/1, Divide/1
  *D/1 -> Gain1/1
  Transfer Fcn1/1 -> Force_Rout/1
  Product/1 -> Sum2/2, Sum3/2, atan(B*β)/1
  atan(B*β)/1 -> Sum2/1
  Sum2/1 -> E*(B*SA-atan(B*SA))/1
  E*(B*SA-atan(B*SA))/1 -> Sum3/1
  "Force_Rout_Pure "/1(Force_Rout_Pure) -> Product2/1, *D/1
  slip rate/1 -> Product/2
  Product2/1 -> Switch/3, Compare To Zero/1
  Constant1/1 -> Switch/1
  Switch/1 -> B/2
  Compare To Zero/1 -> Switch/2
  BCD/1 -> B/1

== system FourWheelSim_base/TractiveSystem/VCM/speedlimit/kph to motor rpm ==
  kph : Inport
  Gear : Gain  Gain=13.75
  to m/s : Gain  Gain=1000/3600
  toTire_rpm : Gain  Gain=60/(2*pi*0.228)
  rpm : Outport  VectorParamsAs1DForOutWhenUnconnected=off
  wires:
  Gear/1 -> rpm/1
  to m/s/1 -> toTire_rpm/1
  toTire_rpm/1 -> Gear/1
  kph/1 -> to m/s/1

== system FourWheelSim_base/4-wheel Vehicle model/comb slip model/comb Fx calc/Force_Fin_comb_FX/Tire Force ==
  Load : Inport
  Slip Rate : Inport  Port=2
  *D*cos(delta) : Product  RndMeth=Zero
  B : Product  Inputs=*/
  BCD : Gain  Gain=afx_f(4)
  C : Constant  Value=afx_f(1)
  Compare To Zero : simulink/Logic and Bit Operations/Compare To Zero  relop===  OutDataTypeStr=boolean
  Constant : Constant  Value=afx_f(3)
  Constant1 : Constant  Value=eps
  D : Product  RndMeth=Zero
  Divide : Product  Inputs=*/
  E*(B*SA-atan(B*SA)) : Product  RndMeth=Zero
  Gain : Gain  Gain=2
  Product : Product  RndMeth=Zero
  Product1 : Product  RndMeth=Zero
  Product2 : Product
  Sum : Sum  Inputs=|++
  Sum1 : Sum  Inputs=|++
  Sum2 : Sum  Inputs=|-+
  Sum3 : Sum  Inputs=|-+
  Switch : Switch  Threshold=0.5
  Trigonometric Function : Trigonometry  Operator=atan
  Trigonometric Function2 : Trigonometry
  a4 : Constant  Value=afx_f(5)
  a5*W : Gain  Gain=afx_f(6)
  a6 : Constant  Value=afx_f(7)
  ai*W : Gain  Gain=afx_f(2)
  atan(B*β) : Trigonometry  Operator=atan
  atan(W/a4) : Trigonometry  Operator=atan
  sin(2*atan(w/a4)) : Trigonometry
  Force_Rear : Outport  VectorParamsAs1DForOutWhenUnconnected=off
  wires:
  Constant/1 -> Sum/2
  ai*W/1 -> Sum/1
  Sum/1 -> D/1
  a4/1 -> Divide/2
  Divide/1 -> atan(W/a4)/1
  atan(W/a4)/1 -> Gain/1
  Gain/1 -> sin(2*atan(w/a4))/1
  sin(2*atan(w/a4))/1 -> BCD/1
  BCD/1 -> B/1
  C/1 -> Product1/2, Product2/2
  a5*W/1 -> Sum1/1
  a6/1 -> Sum1/2
  B/1 -> Product/1
  Slip Rate/1 -> Product/2
  Sum1/1 -> E*(B*SA-atan(B*SA))/2
  Sum3/1 -> Trigonometric Function/1
  D/1 -> Product2/1, *D*cos(delta)/1
  Trigonometric Function/1 -> Product1/1
  Trigonometric Function2/1 -> *D*cos(delta)/2
  Product1/1 -> Trigonometric Function2/1
  Load/1 -> a5*W/1, Divide/1, D/2, ai*W/1
  Product2/1 -> Switch/3, Compare To Zero/1
  Compare To Zero/1 -> Switch/2
  Constant1/1 -> Switch/1
  Switch/1 -> B/2
  *D*cos(delta)/1 -> Force_Rear/1
  Product/1 -> Sum2/2, Sum3/2, atan(B*β)/1
  atan(B*β)/1 -> Sum2/1
  Sum2/1 -> E*(B*SA-atan(B*SA))/1
  E*(B*SA-atan(B*SA))/1 -> Sum3/1

== system FourWheelSim_base/4-wheel Vehicle model/comb slip model/comb Fx calc/Force_Fout_comb_FX/Tire Force ==
  Load : Inport
  Slip Rate : Inport  Port=2
  *D*cos(delta) : Product  RndMeth=Zero
  B : Product  Inputs=*/
  BCD : Gain  Gain=afx_f(4)
  C : Constant  Value=afx_f(1)
  Compare To Zero : simulink/Logic and Bit Operations/Compare To Zero  relop===  OutDataTypeStr=boolean
  Constant : Constant  Value=afx_f(3)
  Constant1 : Constant  Value=eps
  D : Product  RndMeth=Zero
  Divide : Product  Inputs=*/
  E*(B*SA-atan(B*SA)) : Product  RndMeth=Zero
  Gain : Gain  Gain=2
  Product : Product  RndMeth=Zero
  Product1 : Product  RndMeth=Zero
  Product2 : Product
  Sum : Sum  Inputs=|++
  Sum1 : Sum  Inputs=|++
  Sum2 : Sum  Inputs=|-+
  Sum3 : Sum  Inputs=|-+
  Switch : Switch  Threshold=0.5
  Trigonometric Function : Trigonometry  Operator=atan
  Trigonometric Function2 : Trigonometry
  a4 : Constant  Value=afx_f(5)
  a5*W : Gain  Gain=afx_f(6)
  a6 : Constant  Value=afx_f(7)
  ai*W : Gain  Gain=afx_f(2)
  atan(B*β) : Trigonometry  Operator=atan
  atan(W/a4) : Trigonometry  Operator=atan
  sin(2*atan(w/a4)) : Trigonometry
  Force_Rear : Outport  VectorParamsAs1DForOutWhenUnconnected=off
  wires:
  Constant/1 -> Sum/2
  ai*W/1 -> Sum/1
  Sum/1 -> D/1
  a4/1 -> Divide/2
  Divide/1 -> atan(W/a4)/1
  atan(W/a4)/1 -> Gain/1
  Gain/1 -> sin(2*atan(w/a4))/1
  sin(2*atan(w/a4))/1 -> BCD/1
  BCD/1 -> B/1
  C/1 -> Product1/2, Product2/2
  a5*W/1 -> Sum1/1
  a6/1 -> Sum1/2
  B/1 -> Product/1
  Slip Rate/1 -> Product/2
  Sum1/1 -> E*(B*SA-atan(B*SA))/2
  Sum3/1 -> Trigonometric Function/1
  D/1 -> Product2/1, *D*cos(delta)/1
  Trigonometric Function/1 -> Product1/1
  Trigonometric Function2/1 -> *D*cos(delta)/2
  Product1/1 -> Trigonometric Function2/1
  Load/1 -> a5*W/1, Divide/1, D/2, ai*W/1
  Product2/1 -> Switch/3, Compare To Zero/1
  Compare To Zero/1 -> Switch/2
  Constant1/1 -> Switch/1
  Switch/1 -> B/2
  *D*cos(delta)/1 -> Force_Rear/1
  Product/1 -> Sum2/2, Sum3/2, atan(B*β)/1
  atan(B*β)/1 -> Sum2/1
  Sum2/1 -> E*(B*SA-atan(B*SA))/1
  E*(B*SA-atan(B*SA))/1 -> Sum3/1

== system FourWheelSim_base/4-wheel Vehicle model/comb slip model/comb Fx calc/Force_Rin_comb_FX/Tire Force ==
  Load : Inport
  Slip Rate : Inport  Port=2
  *D*cos(delta) : Product  RndMeth=Zero
  B : Product  Inputs=*/
  BCD : Gain  Gain=afx_r(4)
  C : Constant  Value=afx_r(1)
  Compare To Zero : simulink/Logic and Bit Operations/Compare To Zero  relop===  OutDataTypeStr=boolean
  Constant : Constant  Value=afx_r(3)
  Constant1 : Constant  Value=eps
  D : Product  RndMeth=Zero
  Divide : Product  Inputs=*/
  E*(B*SA-atan(B*SA)) : Product  RndMeth=Zero
  Gain : Gain  Gain=2
  Product : Product  RndMeth=Zero
  Product1 : Product  RndMeth=Zero
  Product2 : Product
  Sum : Sum  Inputs=|++
  Sum1 : Sum  Inputs=|++
  Sum2 : Sum  Inputs=|-+
  Sum3 : Sum  Inputs=|-+
  Switch : Switch  Threshold=0.5
  Trigonometric Function : Trigonometry  Operator=atan
  Trigonometric Function2 : Trigonometry
  a4 : Constant  Value=afx_r(5)
  a5*W : Gain  Gain=afx_r(6)
  a6 : Constant  Value=afx_r(7)
  ai*W : Gain  Gain=afx_r(2)
  atan(B*β) : Trigonometry  Operator=atan
  atan(W/a4) : Trigonometry  Operator=atan
  sin(2*atan(w/a4)) : Trigonometry
  Force_Rear : Outport  VectorParamsAs1DForOutWhenUnconnected=off
  wires:
  Constant/1 -> Sum/2
  ai*W/1 -> Sum/1
  Sum/1 -> D/1
  a4/1 -> Divide/2
  Divide/1 -> atan(W/a4)/1
  atan(W/a4)/1 -> Gain/1
  Gain/1 -> sin(2*atan(w/a4))/1
  sin(2*atan(w/a4))/1 -> BCD/1
  BCD/1 -> B/1
  C/1 -> Product1/2, Product2/2
  a5*W/1 -> Sum1/1
  a6/1 -> Sum1/2
  B/1 -> Product/1
  Slip Rate/1 -> Product/2
  Sum1/1 -> E*(B*SA-atan(B*SA))/2
  Sum3/1 -> Trigonometric Function/1
  D/1 -> Product2/1, *D*cos(delta)/1
  Trigonometric Function/1 -> Product1/1
  Trigonometric Function2/1 -> *D*cos(delta)/2
  Product1/1 -> Trigonometric Function2/1
  Load/1 -> a5*W/1, Divide/1, D/2, ai*W/1
  Product2/1 -> Switch/3, Compare To Zero/1
  Compare To Zero/1 -> Switch/2
  Constant1/1 -> Switch/1
  Switch/1 -> B/2
  *D*cos(delta)/1 -> Force_Rear/1
  Product/1 -> Sum2/2, Sum3/2, atan(B*β)/1
  atan(B*β)/1 -> Sum2/1
  Sum2/1 -> E*(B*SA-atan(B*SA))/1
  E*(B*SA-atan(B*SA))/1 -> Sum3/1

== system FourWheelSim_base/4-wheel Vehicle model/comb slip model/comb Fx calc/Force_Rout_comb1_FX/Tire Force ==
  Load : Inport
  Slip Rate : Inport  Port=2
  *D*cos(delta) : Product  RndMeth=Zero
  B : Product  Inputs=*/
  BCD : Gain  Gain=afx_r(4)
  C : Constant  Value=afx_r(1)
  Compare To Zero : simulink/Logic and Bit Operations/Compare To Zero  relop===  OutDataTypeStr=boolean
  Constant : Constant  Value=afx_r(3)
  Constant1 : Constant  Value=eps
  D : Product  RndMeth=Zero
  Divide : Product  Inputs=*/
  E*(B*SA-atan(B*SA)) : Product  RndMeth=Zero
  Gain : Gain  Gain=2
  Product : Product  RndMeth=Zero
  Product1 : Product  RndMeth=Zero
  Product2 : Product
  Sum : Sum  Inputs=|++
  Sum1 : Sum  Inputs=|++
  Sum2 : Sum  Inputs=|-+
  Sum3 : Sum  Inputs=|-+
  Switch : Switch  Threshold=0.5
  Trigonometric Function : Trigonometry  Operator=atan
  Trigonometric Function2 : Trigonometry
  a4 : Constant  Value=afx_r(5)
  a5*W : Gain  Gain=afx_r(6)
  a6 : Constant  Value=afx_r(7)
  ai*W : Gain  Gain=afx_r(2)
  atan(B*β) : Trigonometry  Operator=atan
  atan(W/a4) : Trigonometry  Operator=atan
  sin(2*atan(w/a4)) : Trigonometry
  Force_Rear : Outport  VectorParamsAs1DForOutWhenUnconnected=off
  wires:
  Constant/1 -> Sum/2
  ai*W/1 -> Sum/1
  Sum/1 -> D/1
  a4/1 -> Divide/2
  Divide/1 -> atan(W/a4)/1
  atan(W/a4)/1 -> Gain/1
  Gain/1 -> sin(2*atan(w/a4))/1
  sin(2*atan(w/a4))/1 -> BCD/1
  BCD/1 -> B/1
  C/1 -> Product1/2, Product2/2
  a5*W/1 -> Sum1/1
  a6/1 -> Sum1/2
  B/1 -> Product/1
  Slip Rate/1 -> Product/2
  Sum1/1 -> E*(B*SA-atan(B*SA))/2
  Sum3/1 -> Trigonometric Function/1
  D/1 -> Product2/1, *D*cos(delta)/1
  Trigonometric Function/1 -> Product1/1
  Trigonometric Function2/1 -> *D*cos(delta)/2
  Product1/1 -> Trigonometric Function2/1
  Load/1 -> a5*W/1, Divide/1, D/2, ai*W/1
  Product2/1 -> Switch/3, Compare To Zero/1
  Compare To Zero/1 -> Switch/2
  Constant1/1 -> Switch/1
  Switch/1 -> B/2
  *D*cos(delta)/1 -> Force_Rear/1
  Product/1 -> Sum2/2, Sum3/2, atan(B*β)/1
  atan(B*β)/1 -> Sum2/1
  Sum2/1 -> E*(B*SA-atan(B*SA))/1
  E*(B*SA-atan(B*SA))/1 -> Sum3/1

== system FourWheelSim_base/4-wheel Vehicle model/comb slip model/comb Fy calc/Force_Fin_comb_FY/Force_Fin_Pure ==
  W_Fin : Inport
  beta_Fin : Inport  Port=2
  *D*cos(delta) : Product  RndMeth=Zero
  B : Product  Inputs=*/
  B*β : Product  Inputs=**
  BCD : Gain  Gain=a_f(4)
  C : Constant  Value=a_f(1)
  Compare To Zero : simulink/Logic and Bit Operations/Compare To Zero  relop===  OutDataTypeStr=boolean
  Constant : Constant  Value=a_f(3)
  Constant1 : Constant  Value=eps
  D : Product  RndMeth=Zero
  Divide : Product  Inputs=*/
  E*(B*SA-atan(B*SA)) : Product  RndMeth=Zero
  Gain : Gain  Gain=2
  Product : Product  RndMeth=Zero
  Product1 : Product  RndMeth=Zero
  Product2 : Product
  Sum : Sum  Inputs=|++
  Sum1 : Sum  Inputs=|++
  Sum2 : Sum  Inputs=|-+
  Sum3 : Sum  Inputs=|-+
  Switch : Switch  Threshold=0.5
  Trigonometric Function : Trigonometry  Operator=atan
  Trigonometric Function2 : Trigonometry
  a4 : Constant  Value=a_f(5)
  a5*W : Gain  Gain=a_f(6)
  a6 : Constant  Value=a_f(7)
  ai*W : Gain  Gain=a_f(2)
  atan(B*β) : Trigonometry  Operator=atan
  atan(W/a4) : Trigonometry  Operator=atan
  sin(2*atan(w/a4)) : Trigonometry
  Force_Fin_Pure : Outport  VectorParamsAs1DForOutWhenUnconnected=off
  wires:
  Constant/1 -> Sum/2
  ai*W/1 -> Sum/1
  Sum/1 -> D/1
  a4/1 -> Divide/2
  Divide/1 -> atan(W/a4)/1
  atan(W/a4)/1 -> Gain/1
  Gain/1 -> sin(2*atan(w/a4))/1
  sin(2*atan(w/a4))/1 -> BCD/1
  BCD/1 -> B/1
  C/1 -> Product1/2, Product2/2
  a5*W/1 -> Sum1/1
  a6/1 -> Sum1/2
  B/1 -> Product/1
  beta_Fin/1 -> Product/2
  Sum1/1 -> E*(B*SA-atan(B*SA))/2
  Sum3/1 -> Trigonometric Function/1
  D/1 -> Product2/1, *D*cos(delta)/1
  Trigonometric Function/1 -> Product1/1
  Trigonometric Function2/1 -> *D*cos(delta)/2
  Product1/1 -> Trigonometric Function2/1
  W_Fin/1 -> a5*W/1, Divide/1, D/2, ai*W/1
  Product2/1 -> Switch/3, Compare To Zero/1
  Compare To Zero/1 -> Switch/2
  Constant1/1 -> Switch/1
  Switch/1 -> B/2
  *D*cos(delta)/1 -> Force_Fin_Pure/1
  Product/1 -> Sum2/2, Sum3/2, atan(B*β)/1
  atan(B*β)/1 -> Sum2/1
  Sum2/1 -> E*(B*SA-atan(B*SA))/1
  E*(B*SA-atan(B*SA))/1 -> Sum3/1

== system FourWheelSim_base/4-wheel Vehicle model/comb slip model/comb Fy calc/Force_Fout_comb_FY/Force_Fout_Pure ==
  W_Fin : Inport
  beta_Fin : Inport  Port=2
  *D*cos(delta) : Product  RndMeth=Zero
  B : Product  Inputs=*/
  B*β : Product  Inputs=**
  BCD : Gain  Gain=a_f(4)
  C : Constant  Value=a_f(1)
  Compare To Zero : simulink/Logic and Bit Operations/Compare To Zero  relop===  OutDataTypeStr=boolean
  Constant : Constant  Value=a_f(3)
  Constant1 : Constant  Value=eps
  D : Product  RndMeth=Zero
  Divide : Product  Inputs=*/
  E*(B*SA-atan(B*SA)) : Product  RndMeth=Zero
  Gain : Gain  Gain=2
  Product : Product  RndMeth=Zero
  Product1 : Product  RndMeth=Zero
  Product2 : Product
  Sum : Sum  Inputs=|++
  Sum1 : Sum  Inputs=|++
  Sum2 : Sum  Inputs=|-+
  Sum3 : Sum  Inputs=|-+
  Switch : Switch  Threshold=0.5
  Trigonometric Function : Trigonometry  Operator=atan
  Trigonometric Function2 : Trigonometry
  a4 : Constant  Value=a_f(5)
  a5*W : Gain  Gain=a_f(6)
  a6 : Constant  Value=a_f(7)
  ai*W : Gain  Gain=a_f(2)
  atan(B*β) : Trigonometry  Operator=atan
  atan(W/a4) : Trigonometry  Operator=atan
  sin(2*atan(w/a4)) : Trigonometry
  Force_Fout_Pure : Outport  VectorParamsAs1DForOutWhenUnconnected=off
  wires:
  Constant/1 -> Sum/2
  ai*W/1 -> Sum/1
  Sum/1 -> D/1
  a4/1 -> Divide/2
  Divide/1 -> atan(W/a4)/1
  atan(W/a4)/1 -> Gain/1
  Gain/1 -> sin(2*atan(w/a4))/1
  sin(2*atan(w/a4))/1 -> BCD/1
  BCD/1 -> B/1
  C/1 -> Product1/2, Product2/2
  a5*W/1 -> Sum1/1
  a6/1 -> Sum1/2
  B/1 -> Product/1
  beta_Fin/1 -> Product/2
  Sum1/1 -> E*(B*SA-atan(B*SA))/2
  Sum3/1 -> Trigonometric Function/1
  D/1 -> Product2/1, *D*cos(delta)/1
  Trigonometric Function/1 -> Product1/1
  Trigonometric Function2/1 -> *D*cos(delta)/2
  Product1/1 -> Trigonometric Function2/1
  W_Fin/1 -> a5*W/1, Divide/1, D/2, ai*W/1
  Product2/1 -> Switch/3, Compare To Zero/1
  Compare To Zero/1 -> Switch/2
  Constant1/1 -> Switch/1
  Switch/1 -> B/2
  *D*cos(delta)/1 -> Force_Fout_Pure/1
  Product/1 -> Sum2/2, Sum3/2, atan(B*β)/1
  atan(B*β)/1 -> Sum2/1
  Sum2/1 -> E*(B*SA-atan(B*SA))/1
  E*(B*SA-atan(B*SA))/1 -> Sum3/1

== system FourWheelSim_base/4-wheel Vehicle model/comb slip model/comb Fy calc/Force_Rin_comb_FY/Force_Rin_Pure  ==
  W_Fin : Inport
  beta_Fin : Inport  Port=2
  *D*cos(delta) : Product  RndMeth=Zero
  B : Product  Inputs=*/
  B*β : Product  Commented=on  Inputs=**
  BCD : Gain  Gain=a_r(4)
  C : Constant  Value=a_r(1)
  Compare To Zero : simulink/Logic and Bit Operations/Compare To Zero  relop===  OutDataTypeStr=boolean
  Constant : Constant  Value=a_r(3)
  Constant1 : Constant  Value=eps
  D : Product  RndMeth=Zero
  Divide : Product  Inputs=*/
  E*(B*SA-atan(B*SA)) : Product  RndMeth=Zero
  Gain : Gain  Gain=2
  Product : Product  RndMeth=Zero
  Product1 : Product  RndMeth=Zero
  Product2 : Product
  Sum : Sum  Inputs=|++
  Sum1 : Sum  Inputs=|++
  Sum2 : Sum  Inputs=|-+
  Sum3 : Sum  Inputs=|-+
  Switch : Switch  Threshold=0.5
  Trigonometric Function : Trigonometry  Operator=atan
  Trigonometric Function2 : Trigonometry
  a4 : Constant  Value=a_r(5)
  a5*W : Gain  Gain=a_r(6)
  a6 : Constant  Value=a_r(7)
  ai*W : Gain  Gain=a_r(2)
  atan(B*β) : Trigonometry  Operator=atan
  atan(W/a4) : Trigonometry  Operator=atan
  sin(2*atan(w/a4)) : Trigonometry
  Force_Rin_Pure : Outport  VectorParamsAs1DForOutWhenUnconnected=off
  wires:
  Constant/1 -> Sum/2
  ai*W/1 -> Sum/1
  Sum/1 -> D/1
  a4/1 -> Divide/2
  Divide/1 -> atan(W/a4)/1
  atan(W/a4)/1 -> Gain/1
  Gain/1 -> sin(2*atan(w/a4))/1
  sin(2*atan(w/a4))/1 -> BCD/1
  BCD/1 -> B/1
  C/1 -> Product1/2, Product2/2
  a5*W/1 -> Sum1/1
  a6/1 -> Sum1/2
  B/1 -> Product/1
  beta_Fin/1 -> Product/2
  Sum1/1 -> E*(B*SA-atan(B*SA))/2
  Sum3/1 -> Trigonometric Function/1
  D/1 -> Product2/1, *D*cos(delta)/1
  Trigonometric Function/1 -> Product1/1
  Trigonometric Function2/1 -> *D*cos(delta)/2
  Product1/1 -> Trigonometric Function2/1
  W_Fin/1 -> a5*W/1, Divide/1, D/2, ai*W/1
  Product2/1 -> Switch/3, Compare To Zero/1
  Compare To Zero/1 -> Switch/2
  Constant1/1 -> Switch/1
  Switch/1 -> B/2
  *D*cos(delta)/1 -> Force_Rin_Pure/1
  Product/1 -> Sum2/2, Sum3/2, atan(B*β)/1
  atan(B*β)/1 -> Sum2/1
  Sum2/1 -> E*(B*SA-atan(B*SA))/1
  E*(B*SA-atan(B*SA))/1 -> Sum3/1

== system FourWheelSim_base/4-wheel Vehicle model/comb slip model/comb Fy calc/Force_Rout_comb_FY/Force_Rout_Pure  ==
  W_Fin : Inport
  beta_Fin : Inport  Port=2
  *D*cos(delta) : Product  RndMeth=Zero
  B : Product  Inputs=*/
  B*β : Product  Inputs=**
  BCD : Gain  Gain=a_r(4)
  C : Constant  Value=a_r(1)
  Compare To Zero : simulink/Logic and Bit Operations/Compare To Zero  relop===  OutDataTypeStr=boolean
  Constant : Constant  Value=a_r(3)
  Constant1 : Constant  Value=eps
  D : Product  RndMeth=Zero
  Divide : Product  Inputs=*/
  E*(B*SA-atan(B*SA)) : Product  RndMeth=Zero
  Gain : Gain  Gain=2
  Product : Product  RndMeth=Zero
  Product1 : Product  RndMeth=Zero
  Product2 : Product
  Sum : Sum  Inputs=|++
  Sum1 : Sum  Inputs=|++
  Sum2 : Sum  Inputs=|-+
  Sum3 : Sum  Inputs=|-+
  Switch : Switch  Threshold=0.5
  Trigonometric Function : Trigonometry  Operator=atan
  Trigonometric Function2 : Trigonometry
  a4 : Constant  Value=a_r(5)
  a5*W : Gain  Gain=a_r(6)
  a6 : Constant  Value=a_r(7)
  ai*W : Gain  Gain=a_r(2)
  atan(B*β) : Trigonometry  Operator=atan
  atan(W/a4) : Trigonometry  Operator=atan
  sin(2*atan(w/a4)) : Trigonometry
  Force_Rout_Pure : Outport  VectorParamsAs1DForOutWhenUnconnected=off
  wires:
  Constant/1 -> Sum/2
  ai*W/1 -> Sum/1
  Sum/1 -> D/1
  a4/1 -> Divide/2
  Divide/1 -> atan(W/a4)/1
  atan(W/a4)/1 -> Gain/1
  Gain/1 -> sin(2*atan(w/a4))/1
  sin(2*atan(w/a4))/1 -> BCD/1
  BCD/1 -> B/1
  C/1 -> Product1/2, Product2/2
  a5*W/1 -> Sum1/1
  a6/1 -> Sum1/2
  B/1 -> Product/1
  beta_Fin/1 -> Product/2
  Sum1/1 -> E*(B*SA-atan(B*SA))/2
  Sum3/1 -> Trigonometric Function/1
  D/1 -> Product2/1, *D*cos(delta)/1
  Trigonometric Function/1 -> Product1/1
  Trigonometric Function2/1 -> *D*cos(delta)/2
  Product1/1 -> Trigonometric Function2/1
  W_Fin/1 -> a5*W/1, Divide/1, D/2, ai*W/1
  Product2/1 -> Switch/3, Compare To Zero/1
  Compare To Zero/1 -> Switch/2
  Constant1/1 -> Switch/1
  Switch/1 -> B/2
  *D*cos(delta)/1 -> Force_Rout_Pure/1
  Product/1 -> Sum2/2, Sum3/2, atan(B*β)/1
  atan(B*β)/1 -> Sum2/1
  Sum2/1 -> E*(B*SA-atan(B*SA))/1
  E*(B*SA-atan(B*SA))/1 -> Sum3/1
